simulink model "SetResetWait"  (Simulink 5.0)
settings: Solver=ode45  StartTime=0.0  StopTime=10.0  RelTol=1e-3
settings Model: Creator=scaife  LastModifiedBy=scaife  ExtModeAutoUpdateStatusClock=off

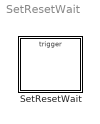
== system SetResetWait ==
  SetResetWait : Stateflow chart

== stateflow chart SetResetWait ==
  state On
  state Off
  state Wait
  On -> Wait : Suspend
  On -> Off : Reset
  Off -> On : Set
  Off -> Wait : Suspend
  Wait -> Off : Clear
  (default) -> Off
  events: Clear input EITHER_EDGE_EVENT; Reset input EITHER_EDGE_EVENT; Suspend input EITHER_EDGE_EVENT; Set input EITHER_EDGE_EVENT
